simulink model "Log10Base"  (R2021b)
settings: Solver=VariableStepAuto  StartTime=0.0  StopTime=10.0  RelTol=1e-3
InitFcn:
  | f = 12.288e6;
  | fs = 153.6e6;
  | N = 2048;
  | n = 0:N-1;
  | Hamming = 0.54 + 0.46 * cos(2*pi*n/N);
  | Hanning = 0.5 * (1 + cos(2*pi*n/N));
  | Norm_Ham = sum(Hamming);
  | Norm_Han = sum(Hanning);
libraries: hlsMath x1, vmcUtilities x1
settings Model: Creator=yxb20126  LastModifiedBy=yxb20126

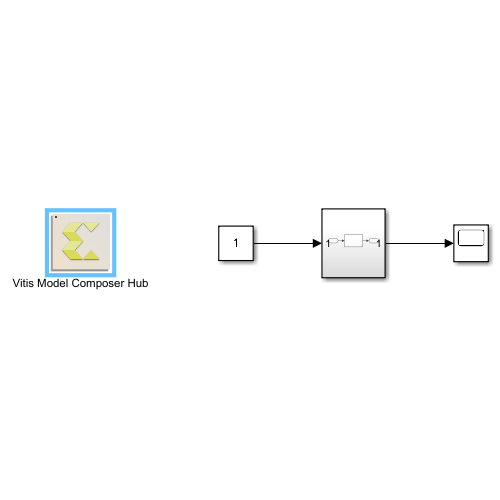
[thumbnail: Simulink's stored preview of the top-level diagram]
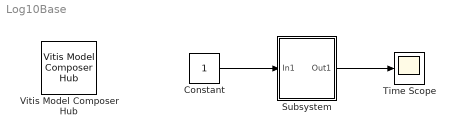
== system Log10Base ==
  Constant : Constant  SampleTime=1/fs
  Subsystem : Subsystem
  Time Scope : Scope
  Vitis Model Composer Hub : vmcUtilities/Vitis Model Composer Hub  Tag=genX  CodeGeneration=off  SubsystemName=Subsystem  TargetDirectory=H:/19496/STFT/Log  ExportType=IP Catalog  IpVendor=xilinx.com  IpLibrary=hls  IpName=Log10Base  IpVersion=1.0  IpHWLanguage=Verilog  AieCompilerOptions={}  CreateTestbench=on  TestbenchStackSize=10  RunAieSim=off  AieSimTimeout=50000  RunAieSimProfiling=off  LaunchVitisAnalyzer=off  PlotOutput=off  RunX86Sim=off  X86SimTimeout=10  GenHwImage=off  PlatformType=Not Specified  HwSystemType=Baremetal  HwValidationTarget=hw  ProjDevice=xczu48dr-ffvg1517-2-e  ProjDevicePart=xczu48dr-ffvg1517-2-e  SamplePeriod=-1  ClockFrequency=200  DataPathParallelism=1  xilinxfamily=zynquplusRFSOC  part=xczu48dr  speed=-2-e  package=ffvg1517  directory=./netlist  testbench=off  incr_netlist=off  synthesis_tool=Vivado  clock_wrapper=Clock Enables  dbl_ovrd=According to Block Masks  dcm_input_clock_period=10  sysclk_period=(1/fs)*10e9  simulink_period=1/fs  eval_field=0
  wires:
  Subsystem/1(Out1) -> Time Scope/1
  Constant/1 -> Subsystem/1(In1)

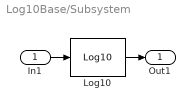
== system Log10Base/Subsystem ==
  In1 : Inport
  Log10 : hlsMath/Log10
  Out1 : Outport
  wires:
  In1/1 -> Log10/1
  Log10/1 -> Out1/1
